simulink model "btp2"  (R2022a)
settings: Solver=ode45  StartTime=0.0  StopTime=inf  RelTol=1e-3  EnableMultiTasking=on
libraries: rllib x1
settings Model: Creator=sneha  LastModifiedBy=archi
settings SolverCC: AlgebraicLoopSolver=TrustRegion
settings DataIOCC: LimitDataPoints=on  SaveFormat=Array
settings OptimizationCC: LifeSpan=inf
settings DebuggingCC: UnconnectedInputMsg=warning  UnconnectedOutputMsg=warning  UnconnectedLineMsg=warning  SFUnexpectedBacktrackingDiag=warning  SFNoUnconditionalDefaultTransitionDiag=warning  SFExecutionAtInitializationDiag=none  SFMachineParentedDataDiag=warning  ArithmeticOperatorsInVariantConditions=warning
settings HardwareCC: ProdBitPerPointer=32  ProdBitPerSizeT=32  ProdBitPerPtrDiffT=32  ProdLargestAtomicFloat=None  ProdIntDivRoundTo=Undefined  ProdEndianess=Unspecified  ProdWordSize=32  ProdHWDeviceType=32-bit Generic
settings ModelReferenceCC: PropagateSignalLabelsOutOfModel=off
settings SFSimCC: SimUseLocalCustomCode=off  CustomCodeUndefinedFunction=UseInterfaceOnly
settings RTWCC: RTWUseLocalCustomCode=off
settings CodeAppCC: StateflowObjectComments=on
settings GRTTargetCC: TargetLangStandard=C89/C90 (ANSI)
settings ConfigComp: CovMetricSettings=dw  CovSaveCumulativeToWorkspaceVar=on  CovSaveSingleToWorkspaceVar=on  CovExternalEMLEnable=off

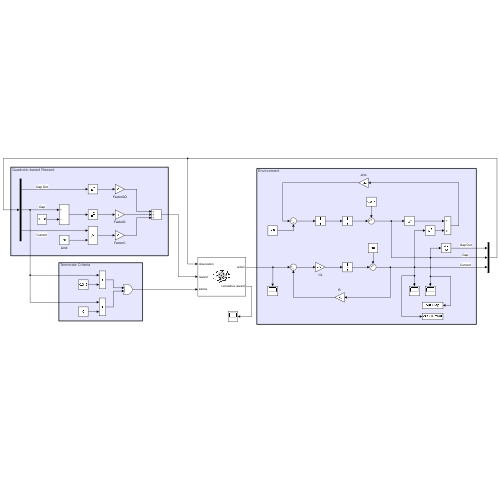
[thumbnail: Simulink's stored preview of the top-level diagram]
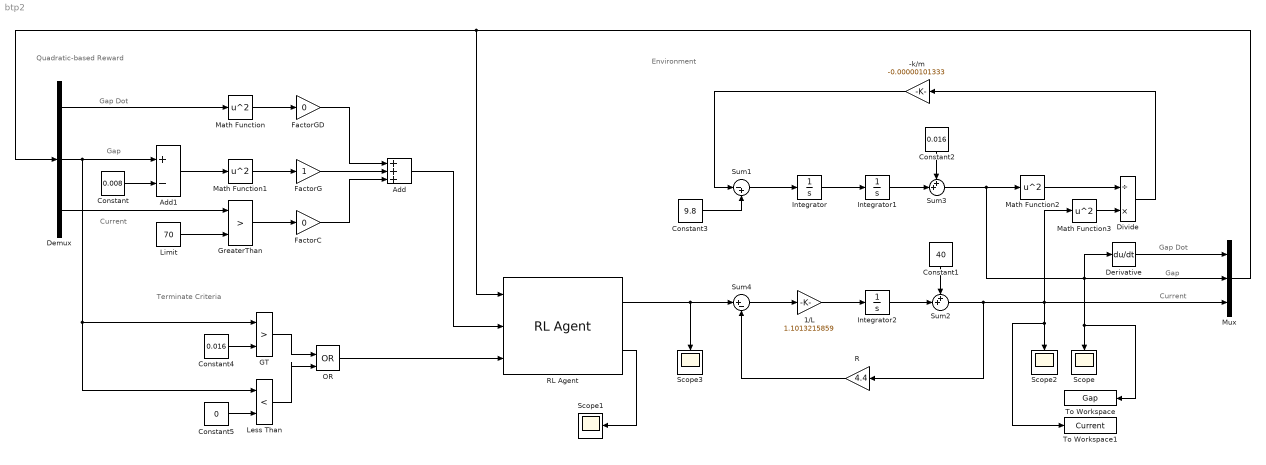
== system btp2 ==
  note: Terminate Criteria
  note: Quadratic-based Reward
  note: Gap Dot
  note: Current
  note: Gap
  note: Environment
  note: Current
  note: Gap
  note: Gap Dot
  -k/m : Gain  Gain=-0.00000101333
  1/L : Gain  Gain=1.1013215859
  Add : Sum  Inputs=+++
  Add1 : Sum  Inputs=+-
  Constant : Constant  Value=0.008
  Constant1 : Constant  Value=40
  Constant2 : Constant  Value=0.016
  Constant3 : Constant  Value=9.8
  Constant4 : Constant  Value=0.016
  Constant5 : Constant  Value=0
  Demux : Demux  Outputs=3
  Derivative : Derivative
  Divide : Product  Inputs=/*
  FactorC : Gain  Gain=0
  FactorG : Gain
  FactorGD : Gain  Gain=0
  GT : RelationalOperator  Operator=>  OutDataTypeStr=boolean  RndMeth=Simplest  InputSameDT=off
  GreaterThan : RelationalOperator  Operator=>  OutDataTypeStr=boolean  RndMeth=Simplest  InputSameDT=off
  Integrator : Integrator
  Integrator1 : Integrator
  Integrator2 : Integrator
  Less Than : RelationalOperator  Operator=<  OutDataTypeStr=boolean  RndMeth=Simplest  InputSameDT=off
  Limit : Constant  Value=70
  Math Function{,1..3} (4 alike) : Math  Operator=square
  Mux : Mux  Inputs=3
  OR : Logic  Operator=OR  IconShape=distinctive  AllPortsSameDT=off  OutDataTypeStr=boolean
  R : Gain  Gain=4.4
  RL Agent : rllib/RL Agent  Agent=rlDDPGAgent  ExternalActionAsInput=off  ProvideLastAction=off  ProvideCumRwd=on  TreatAsDirectFeedthrough=on  UseStrictObservationDataTypes=off
  Scope{,1..3} (4 alike) : Scope
  Sum1 : Sum  Inputs=|-+
  Sum2 : Sum  Inputs=++|
  Sum3 : Sum  Inputs=++|
  Sum4 : Sum  Inputs=|+-
  To Workspace : ToWorkspace  VariableName=Gap  SaveFormat=Timeseries  SampleTime=-1
  To Workspace1 : ToWorkspace  VariableName=Current  SaveFormat=Timeseries  SampleTime=-1
  wires:
  Math Function2/1 -> Divide/1
  Sum1/1 -> Integrator/1
  Math Function3/1 -> Divide/2
  -k/m/1 -> Sum1/1
  R/1 -> Sum4/2
  1/L/1 -> Integrator2/1
  Integrator/1 -> Integrator1/1
  Sum4/1 -> 1/L/1
  Divide/1 -> -k/m/1
  Constant3/1 -> Sum1/2
  Integrator2/1 -> Sum2/2
  Sum2/1 -> R/1, Math Function3/1, To Workspace1/1, Scope2/1, Mux/3
  Constant2/1 -> Sum3/1
  Integrator1/1 -> Sum3/2
  Constant1/1 -> Sum2/1
  Sum3/1 -> Math Function2/1, Derivative/1, Scope/1, To Workspace/1, Mux/2
  RL Agent/1 -> Scope3/1, Sum4/1
  Derivative/1 -> Mux/1
  Add/1 -> RL Agent/2
  Mux/1 -> RL Agent/1, Demux/1
  Math Function1/1 -> FactorG/1
  FactorGD/1 -> Add/1
  Math Function/1 -> FactorGD/1
  Demux/3 -> GreaterThan/1
  Limit/1 -> GreaterThan/2
  GreaterThan/1 -> FactorC/1
  FactorG/1 -> Add/2
  Demux/1 -> Math Function/1
  FactorC/1 -> Add/3
  Constant/1 -> Add1/2
  Add1/1 -> Math Function1/1
  OR/1 -> RL Agent/3
  Demux/2 -> Less Than/1, GT/1, Add1/1
  GT/1 -> OR/1
  Constant4/1 -> GT/2
  Less Than/1 -> OR/2
  Constant5/1 -> Less Than/2
  RL Agent/2 -> Scope1/1
